simulink library "eng_simple_transient_std"  (Simulink 8.7)
settings: Solver=ode45  StartTime=0.0  StopTime=10.0  RelTol=1e-3
undefined symbols (not defined in the file): DiscIntNeverNeededParam, sMP
libraries: simulink x17
(part 3 of 3)

== system eng_simple_transient_std/eng_simple_transient_std/Airpath_model/Intake flows calculation/EGRTAT filter ==
  EGRTAT_sp : Inport
  Constant : Constant
  Digital Clock : DigitalClock  SampleTime=-1
  Fcn : Fcn  Expr=u(2)/(u(2)+u(1))
  Initialisation : Switch  Criteria=u2 > Threshold
  Lookup Table : Lookup  InputValues=Fiter_calibration_fmode_x_NMOT_rpm  Table=Fiter_calibration_fmode_y_tc_EGRTAT  LookUpMeth=Interpolation-Use End Values
  Memory4 : Memory  InheritSampleTime=on
  Mux : Mux  Inputs=2
  Product : Product  SaturateOnIntegerOverflow=on  InputSameDT=on  OutDataTypeStr=Inherit: Same as first input
  Product1 : Product  SaturateOnIntegerOverflow=on  InputSameDT=on  OutDataTypeStr=Inherit: Same as first input
  Sum : Sum  Inputs=|+-  SaturateOnIntegerOverflow=on  InputSameDT=on  OutDataTypeStr=Inherit: Same as first input
  Sum1 : Sum  Inputs=|++  SaturateOnIntegerOverflow=on  InputSameDT=on  OutDataTypeStr=Inherit: Same as first input
  dt : Constant  Value=Fiter_calibration_dt
  EGRTAT : Outport
  wires:
  Initialisation/1 -> EGRTAT/1, Memory4/1
  Sum1/1 -> Initialisation/1
  Digital Clock/1 -> Initialisation/2
  Fcn/1 -> Sum/2, Product1/1
  Constant/1 -> Sum/1
  Sum/1 -> Product/2
  Product1/1 -> Sum1/2
  Product/1 -> Sum1/1
  Memory4/1 -> Product/1
  EGRTAT_sp/1 -> Initialisation/3, Product1/2
  dt/1 -> Mux/2
  Lookup Table/1 -> Mux/1
  Mux/1 -> Fcn/1
  [EngSpeed] -> Lookup Table/1

== system eng_simple_transient_std/eng_simple_transient_std/Engine_model/AdBlue consumption/Calc_AdBlue_Consumption ==
  brakingMode : Inport
  MAdBlue_kgh : Inport  Port=2
  MAdBlue_braking : Constant  Value=0
  Multiport Switch1 : MultiPortSwitch  DataPortOrder=Zero-based contiguous  Inputs=5  zeroidx=on
  rpm->rph2 : Gain  Gain=1/2
  MAdBlue_brk_kgh : Outport
  wires:
  MAdBlue_kgh/1 -> Multiport Switch1/6, rpm->rph2/1, Multiport Switch1/2
  MAdBlue_braking/1 -> Multiport Switch1/5
  rpm->rph2/1 -> Multiport Switch1/4, Multiport Switch1/3
  brakingMode/1 -> Multiport Switch1/1
  Multiport Switch1/1 -> MAdBlue_brk_kgh/1

== system eng_simple_transient_std/eng_simple_transient_std/Engine_model/Fuel consumption calculation/Calc_Fuel_Flow ==
  brakingMode : Inport
  Mfuel_mgstr_sp : Inport  Port=2
  Constant : Constant  Value=Eng_characteristics_n_cylinder
  Mfuel_Braking : Constant  Value=0
  Multiport Switch1 : MultiPortSwitch  DataPortOrder=Zero-based contiguous  Inputs=5  zeroidx=on
  Product : Product  RndMeth=Zero
  fuelConsumtion_kgh1 : Product  Inputs=**
  mg_str->kg_rota : Fcn  Expr=u/2/1e6
  rpm->rph1 : Gain  Gain=60
  rpm->rph2 : Gain  Gain=1/2
  MFuel_kgh : Outport
  wires:
  Constant/1 -> Product/1
  Product/1 -> mg_str->kg_rota/1
  Multiport Switch1/1 -> Product/2
  Mfuel_mgstr_sp/1 -> Multiport Switch1/6, rpm->rph2/1, Multiport Switch1/2
  rpm->rph1/1 -> fuelConsumtion_kgh1/2
  mg_str->kg_rota/1 -> fuelConsumtion_kgh1/1
  [EngSpeed] -> rpm->rph1/1
  Mfuel_Braking/1 -> Multiport Switch1/5
  rpm->rph2/1 -> Multiport Switch1/4, Multiport Switch1/3
  brakingMode/1 -> Multiport Switch1/1
  fuelConsumtion_kgh1/1 -> MFuel_kgh/1

== system eng_simple_transient_std/eng_simple_transient_std/Engine_model/Fuel consumption calculation/Calc_Fuel_Flow_Consumption ==
  brakingMode : Inport
  Mfuel_mgstr_sp : Inport  Port=2
  Constant : Constant  Value=Eng_characteristics_n_cylinder
  Mfuel_Braking : Constant  Value=0
  Multiport Switch1 : MultiPortSwitch  DataPortOrder=Zero-based contiguous  Inputs=5  zeroidx=on
  Product : Product  RndMeth=Zero
  fuelConsumtion_kgh1 : Product  Inputs=**
  mg_str->kg_rota : Fcn  Expr=u/2/1e6
  rpm->rph1 : Gain  Gain=60
  rpm->rph2 : Gain  Gain=1/2
  MFuel_kgh : Outport
  wires:
  fuelConsumtion_kgh1/1 -> MFuel_kgh/1
  brakingMode/1 -> Multiport Switch1/1
  rpm->rph2/1 -> Multiport Switch1/3, Multiport Switch1/4
  Mfuel_Braking/1 -> Multiport Switch1/5
  [EngSpeed] -> rpm->rph1/1
  mg_str->kg_rota/1 -> fuelConsumtion_kgh1/1
  rpm->rph1/1 -> fuelConsumtion_kgh1/2
  Mfuel_mgstr_sp/1 -> Multiport Switch1/2, rpm->rph2/1, Multiport Switch1/6
  Multiport Switch1/1 -> Product/2
  Product/1 -> mg_str->kg_rota/1
  Constant/1 -> Product/1

== system eng_simple_transient_std/eng_simple_transient_std/Engine_model/Fuel consumption calculation/Calc_Fuel_Flow_TM1_Consumption ==
  brakingMode : Inport
  Mfuel_mgstr_sp : Inport  Port=2
  Constant : Constant  Value=Eng_characteristics_n_cylinder
  Mfuel_Braking : Constant  Value=0
  Multiport Switch1 : MultiPortSwitch  DataPortOrder=Zero-based contiguous  Inputs=5  zeroidx=on
  Product : Product  RndMeth=Zero
  fuelConsumtion_kgh1 : Product  Inputs=**
  mg_str->kg_rota : Fcn  Expr=u/2/1e6
  rpm->rph1 : Gain  Gain=60
  rpm->rph2 : Gain  Gain=1/2
  MFuel_kgh : Outport
  wires:
  Constant/1 -> Product/1
  Product/1 -> mg_str->kg_rota/1
  Multiport Switch1/1 -> Product/2
  Mfuel_mgstr_sp/1 -> Multiport Switch1/6, rpm->rph2/1, Multiport Switch1/2
  rpm->rph1/1 -> fuelConsumtion_kgh1/2
  mg_str->kg_rota/1 -> fuelConsumtion_kgh1/1
  [EngSpeed] -> rpm->rph1/1
  Mfuel_Braking/1 -> Multiport Switch1/5
  rpm->rph2/1 -> Multiport Switch1/4, Multiport Switch1/3
  brakingMode/1 -> Multiport Switch1/1
  fuelConsumtion_kgh1/1 -> MFuel_kgh/1

== system eng_simple_transient_std/eng_simple_transient_std/Engine_model/Fuel consumption calculation/T2N correction ==
  Constant : Constant
  Product : Product  RndMeth=Zero
  Setpoint_fuelledMode_z_dMFueldT2N : Lookup2D  RowIndex=Setpoint_fuelledMode_y_alphaTorque  ColumnIndex=Setpoint_fuelledMode_x_NMOTW_rpm  Table=Setpoint_fuelledMode_z_dMFueldT2N
  Sum : Sum  Inputs=|+-
  Sum1 : Sum  Inputs=|++
  dMFueldT2N : Outport
  wires:
  [T2N_extern] -> Sum/1
  [T2N_degC_sp] -> Sum/2
  [alphaTorque] -> Setpoint_fuelledMode_z_dMFueldT2N/1
  [EngSpeed] -> Setpoint_fuelledMode_z_dMFueldT2N/2
  Setpoint_fuelledMode_z_dMFueldT2N/1 -> Product/1
  Sum/1 -> Product/2
  Product/1 -> Sum1/1
  Constant/1 -> Sum1/2
  Sum1/1 -> dMFueldT2N/1

== system eng_simple_transient_std/eng_simple_transient_std/Engine_model/Fuel consumption calculation/TWE correction ==
  Constant : Constant
  Product : Product  RndMeth=Zero
  Setpoint_fuelledMode_z_dMFueldTWE : Lookup2D  RowIndex=Setpoint_fuelledMode_y_alphaTorque  ColumnIndex=Setpoint_fuelledMode_x_NMOTW_rpm  Table=Setpoint_fuelledMode_z_dMFueldTWE
  Sum : Sum  Inputs=|+-
  Sum1 : Sum  Inputs=|++
  dMFueldTWE : Outport
  wires:
  Sum1/1 -> dMFueldTWE/1
  Constant/1 -> Sum1/2
  Product/1 -> Sum1/1
  Sum/1 -> Product/2
  Setpoint_fuelledMode_z_dMFueldTWE/1 -> Product/1
  [EngSpeed] -> Setpoint_fuelledMode_z_dMFueldTWE/2
  [alphaTorque] -> Setpoint_fuelledMode_z_dMFueldTWE/1
  [TWE_degC_sp] -> Sum/2
  [eng_CoolantEngineIn_Temperature] -> Sum/1

== system eng_simple_transient_std/eng_simple_transient_std/Outputs/Calc_exhGas/rCO2_calc ==
  AFR : Inport
  haluft : Inport  Port=2
  Constant2 : Constant  Value=0.0325
  Constant3 : Constant  Value=1000
  Constant5 : Constant  Value=0.0725
  Gain1 : Gain  Gain=0.5
  MolH1 : Constant  Value=18.01528
  Product1 : Product  Inputs=***//  RndMeth=Zero
  Product2 : Product  Inputs=*/  RndMeth=Zero
  Stoech_coeff : Constant  Value=Eng_characteristics_Stoech_coeff
  Sum1 : Sum  Inputs=3
  CO2_molfrac : Outport
  wires:
  Constant5/1 -> Product2/1
  Sum1/1 -> Product2/2
  Gain1/1 -> Sum1/2
  Constant2/1 -> Sum1/1
  Product1/1 -> Sum1/3
  AFR/1 -> Product1/2, Gain1/1
  Stoech_coeff/1 -> Product1/3
  MolH1/1 -> Product1/5
  Constant3/1 -> Product1/4
  haluft/1 -> Product1/1
  Product2/1 -> CO2_molfrac/1

== system eng_simple_transient_std/eng_simple_transient_std/Outputs/Calc_exhGas/rH2O_calc ==
  AFR : Inport
  haluft : Inport  Port=2
  Constant2 : Constant  Value=0.0325
  Constant3 : Constant  Value=1000
  Constant5 : Constant  Value=0.065
  Gain : Gain  Gain=0.5
  MolH1 : Constant  Value=18.01528
  Product1 : Product  Inputs=***//  RndMeth=Zero
  Product2 : Product  Inputs=*/  RndMeth=Zero
  Stoech_coeff : Constant  Value=Eng_characteristics_Stoech_coeff
  Sum1 : Sum  Inputs=3
  Sum3 : Sum  Inputs=|++
  rH2O_Abg : Outport
  wires:
  Product2/1 -> rH2O_Abg/1
  Constant5/1 -> Sum3/1
  Sum3/1 -> Product2/1
  Sum1/1 -> Product2/2
  Gain/1 -> Sum1/2
  Constant2/1 -> Sum1/1
  Product1/1 -> Sum3/2, Sum1/3
  AFR/1 -> Product1/2, Gain/1
  Stoech_coeff/1 -> Product1/3
  MolH1/1 -> Product1/5
  Constant3/1 -> Product1/4
  haluft/1 -> Product1/1

== system eng_simple_transient_std/eng_simple_transient_std/Outputs/Calc_exhGas/rO2_calc ==
  AFR : Inport
  haluft : Inport  Port=2
  Constant1 : Constant  Value=0.0325
  Constant2 : Constant
  Constant4 : Constant  Value=1000
  Gain1 : Gain  Gain=0.5
  Gain2 : Gain  Gain=0.105
  Lim 0<x<0.2078 => lambda<100 : Saturate  UpperLimit=0.2078376487  LowerLimit=1e-16  LinearizeAsGain=off  ZeroCross=off
  MolH2 : Constant  Value=18.01528
  Product3 : Product  Inputs=***//  RndMeth=Zero
  Product4 : Product  Inputs=*/  RndMeth=Zero
  Stoech_coeff : Constant  Value=Eng_characteristics_Stoech_coeff
  Sum1 : Sum  Inputs=+-
  Sum2 : Sum  Inputs=3
  rO2_Abg : Outport
  wires:
  Product4/1 -> Lim 0<x<0.2078 => lambda<100/1
  Gain2/1 -> Product4/1
  Sum1/1 -> Gain2/1
  Constant2/1 -> Sum1/2
  Sum2/1 -> Product4/2
  Gain1/1 -> Sum2/2
  Constant1/1 -> Sum2/1
  Product3/1 -> Sum2/3
  AFR/1 -> Product3/2, Gain1/1, Sum1/1
  Stoech_coeff/1 -> Product3/3
  MolH2/1 -> Product3/5
  Constant4/1 -> Product3/4
  haluft/1 -> Product3/1
  Lim 0<x<0.2078 => lambda<100/1 -> rO2_Abg/1

== system eng_simple_transient_std/eng_simple_transient_std/SetPoint_model/Starter model/engStarted actualisation ==
  b_ignition : Inport
  Trigger : TriggerPort  VariantControl=Variant
  EngStarted : Outport
  wires:
  b_ignition/1 -> EngStarted/1

== system eng_simple_transient_std/eng_simple_transient_std/SetPoint_model/Starter model/starter torque filter ==
  starterTorque_sp : Inport
  Constant : Constant
  Fcn : Fcn  Expr=u(2)/(u(2)+u(1))
  Memory4 : Memory  InheritSampleTime=on
  Mux : Mux  Inputs=2
  Product : Product  SaturateOnIntegerOverflow=on  InputSameDT=on  OutDataTypeStr=Inherit: Same as first input
  Product1 : Product  SaturateOnIntegerOverflow=on  InputSameDT=on  OutDataTypeStr=Inherit: Same as first input
  Sum : Sum  Inputs=|+-  SaturateOnIntegerOverflow=on  InputSameDT=on  OutDataTypeStr=Inherit: Same as first input
  Sum1 : Sum  Inputs=|++  SaturateOnIntegerOverflow=on  InputSameDT=on  OutDataTypeStr=Inherit: Same as first input
  dt : Constant  Value=Fiter_calibration_dt
  tc starter : Constant  Value=Eng_starter_time_constant
  starterTorque : Outport
  wires:
  tc starter/1 -> Mux/1
  Sum1/1 -> Memory4/1, starterTorque/1
  Fcn/1 -> Sum/2, Product1/1
  Constant/1 -> Sum/1
  Sum/1 -> Product/2
  Product1/1 -> Sum1/2
  Product/1 -> Sum1/1
  Memory4/1 -> Product/1
  starterTorque_sp/1 -> Product1/2
  dt/1 -> Mux/2
  Mux/1 -> Fcn/1

== system eng_simple_transient_std/eng_simple_transient_std/SetPoint_model/Torque setpoint/Alpha_p2s_Br1 calculation ==
  p2s : Inport
  EngSpeed : Inport  Port=2
  Constant : Constant  Value=1e-6
  Divide : Product  Inputs=*/
  MaxBrakingPressure : Lookup2D  RowIndex=Setpoint_brakingMode1_y_alphaTorque  ColumnIndex=Setpoint_brakingMode1_x_NMOTW_rpm  Table=Setpoint_brakingMode1_z_P2S_mbar
  MinBrakingPressure : Lookup2D  RowIndex=Setpoint_brakingMode1_y_alphaTorque  ColumnIndex=Setpoint_brakingMode1_x_NMOTW_rpm  Table=Setpoint_brakingMode1_z_P2S_mbar
  MinMax : MinMax  Function=max  Inputs=2
  Saturation : Saturate  UpperLimit=1  LowerLimit=0
  Subtract : Sum  Inputs=-+
  Subtract1 : Sum  Inputs=+-
  alpha0 : Constant  Value=0
  alpha1 : Constant
  alpha_p2s_br1 : Outport
  wires:
  Saturation/1 -> alpha_p2s_br1/1
  Subtract1/1 -> Divide/1
  MaxBrakingPressure/1 -> Subtract/2
  MinBrakingPressure/1 -> Subtract1/2, Subtract/1
  p2s/1 -> Subtract1/1
  EngSpeed/1 -> MinBrakingPressure/2, MaxBrakingPressure/2
  alpha1/1 -> MaxBrakingPressure/1
  alpha0/1 -> MinBrakingPressure/1
  Divide/1 -> Saturation/1
  Constant/1 -> MinMax/2
  Subtract/1 -> MinMax/1
  MinMax/1 -> Divide/2

== system eng_simple_transient_std/eng_simple_transient_std/SetPoint_model/Torque setpoint/Alpha_p2s_Br2 calculation ==
  p2s : Inport
  EngSpeed : Inport  Port=2
  Constant : Constant  Value=1e-6
  Divide : Product  Inputs=*/
  MaxBrakingPressure : Lookup2D  RowIndex=Setpoint_brakingMode2_y_alphaTorque  ColumnIndex=Setpoint_brakingMode2_x_NMOTW_rpm  Table=Setpoint_brakingMode2_z_P2S_mbar
  MinBrakingPressure : Lookup2D  RowIndex=Setpoint_brakingMode2_y_alphaTorque  ColumnIndex=Setpoint_brakingMode2_x_NMOTW_rpm  Table=Setpoint_brakingMode2_z_P2S_mbar
  MinMax : MinMax  Function=max  Inputs=2
  Saturation : Saturate  UpperLimit=1  LowerLimit=0
  Subtract : Sum  Inputs=-+
  Subtract1 : Sum  Inputs=+-
  alpha0 : Constant  Value=0
  alpha1 : Constant
  alpha_p2s_br2 : Outport
  wires:
  Saturation/1 -> alpha_p2s_br2/1
  Subtract1/1 -> Divide/1
  MaxBrakingPressure/1 -> Subtract/2
  MinBrakingPressure/1 -> Subtract1/2, Subtract/1
  p2s/1 -> Subtract1/1
  EngSpeed/1 -> MinBrakingPressure/2, MaxBrakingPressure/2
  alpha1/1 -> MaxBrakingPressure/1
  alpha0/1 -> MinBrakingPressure/1
  Divide/1 -> Saturation/1
  Constant/1 -> MinMax/2
  Subtract/1 -> MinMax/1
  MinMax/1 -> Divide/2

== system eng_simple_transient_std/eng_simple_transient_std/SetPoint_model/Torque setpoint/Alpha_p2s_Br3 calculation ==
  p2s : Inport
  EngSpeed : Inport  Port=2
  Constant : Constant  Value=1e-6
  Divide : Product  Inputs=*/
  MaxBrakingPressure : Lookup2D  RowIndex=Setpoint_brakingMode3_y_alphaTorque  ColumnIndex=Setpoint_brakingMode3_x_NMOTW_rpm  Table=Setpoint_brakingMode3_z_P2S_mbar
  MinBrakingPressure : Lookup2D  RowIndex=Setpoint_brakingMode3_y_alphaTorque  ColumnIndex=Setpoint_brakingMode3_x_NMOTW_rpm  Table=Setpoint_brakingMode3_z_P2S_mbar
  MinMax : MinMax  Function=max  Inputs=2
  Saturation : Saturate  UpperLimit=1  LowerLimit=0
  Subtract : Sum  Inputs=-+
  Subtract1 : Sum  Inputs=+-
  alpha0 : Constant  Value=0
  alpha1 : Constant
  alpha_p2s_br3 : Outport
  wires:
  Saturation/1 -> alpha_p2s_br3/1
  Subtract1/1 -> Divide/1
  MaxBrakingPressure/1 -> Subtract/2
  MinBrakingPressure/1 -> Subtract1/2, Subtract/1
  p2s/1 -> Subtract1/1
  EngSpeed/1 -> MinBrakingPressure/2, MaxBrakingPressure/2
  alpha1/1 -> MaxBrakingPressure/1
  alpha0/1 -> MinBrakingPressure/1
  Divide/1 -> Saturation/1
  Constant/1 -> MinMax/2
  Subtract/1 -> MinMax/1
  MinMax/1 -> Divide/2

== system eng_simple_transient_std/eng_simple_transient_std/SetPoint_model/alpha torque calculation/AlphaBr1 calculation ==
  mcm_act_braking_trq : Inport
  EngSpeed : Inport  Port=2
  Constant : Constant  Value=-1e-6
  Divide : Product  Inputs=*/
  MaxBrakingTorque : Lookup2D  RowIndex=Setpoint_brakingMode1_y_alphaTorque  ColumnIndex=Setpoint_brakingMode1_x_NMOTW_rpm  Table=Setpoint_brakingMode1_z_Torque_Nm
  MinBrakingTorque : Lookup2D  RowIndex=Setpoint_brakingMode1_y_alphaTorque  ColumnIndex=Setpoint_brakingMode1_x_NMOTW_rpm  Table=Setpoint_brakingMode1_z_Torque_Nm
  MinMax : MinMax  Inputs=2
  Subtract : Sum  Inputs=-+
  Subtract1 : Sum  Inputs=+-
  alpha0 : Constant  Value=0
  alpha1 : Constant
  alpha_br1 : Outport
  wires:
  Subtract1/1 -> Divide/1
  MaxBrakingTorque/1 -> Subtract/2
  MinBrakingTorque/1 -> Subtract1/2, Subtract/1
  mcm_act_braking_trq/1 -> Subtract1/1
  EngSpeed/1 -> MinBrakingTorque/2, MaxBrakingTorque/2
  alpha1/1 -> MaxBrakingTorque/1
  alpha0/1 -> MinBrakingTorque/1
  Divide/1 -> alpha_br1/1
  Subtract/1 -> MinMax/1
  Constant/1 -> MinMax/2
  MinMax/1 -> Divide/2

== system eng_simple_transient_std/eng_simple_transient_std/SetPoint_model/alpha torque calculation/AlphaBr2 calculation ==
  mcm_act_braking_trq : Inport
  EngSpeed : Inport  Port=2
  Constant : Constant  Value=-1e-6
  Divide : Product  Inputs=*/
  MaxBrakingTorque : Lookup2D  RowIndex=Setpoint_brakingMode2_y_alphaTorque  ColumnIndex=Setpoint_brakingMode2_x_NMOTW_rpm  Table=Setpoint_brakingMode2_z_Torque_Nm
  MinBrakingTorque : Lookup2D  RowIndex=Setpoint_brakingMode2_y_alphaTorque  ColumnIndex=Setpoint_brakingMode2_x_NMOTW_rpm  Table=Setpoint_brakingMode2_z_Torque_Nm
  MinMax : MinMax  Inputs=2
  Subtract : Sum  Inputs=-+
  Subtract1 : Sum  Inputs=+-
  alpha0 : Constant  Value=0
  alpha1 : Constant
  alpha_br2 : Outport
  wires:
  Divide/1 -> alpha_br2/1
  alpha0/1 -> MinBrakingTorque/1
  alpha1/1 -> MaxBrakingTorque/1
  EngSpeed/1 -> MaxBrakingTorque/2, MinBrakingTorque/2
  mcm_act_braking_trq/1 -> Subtract1/1
  MinBrakingTorque/1 -> Subtract/1, Subtract1/2
  MaxBrakingTorque/1 -> Subtract/2
  Subtract1/1 -> Divide/1
  Constant/1 -> MinMax/2
  Subtract/1 -> MinMax/1
  MinMax/1 -> Divide/2

== system eng_simple_transient_std/eng_simple_transient_std/SetPoint_model/alpha torque calculation/AlphaBr3 calculation ==
  mcm_act_braking_trq : Inport
  EngSpeed : Inport  Port=2
  Constant : Constant  Value=-1e-6
  Divide : Product  Inputs=*/
  MaxBrakingTorque : Lookup2D  RowIndex=Setpoint_brakingMode3_y_alphaTorque  ColumnIndex=Setpoint_brakingMode3_x_NMOTW_rpm  Table=Setpoint_brakingMode3_z_Torque_Nm
  MinBrakingTorque : Lookup2D  RowIndex=Setpoint_brakingMode3_y_alphaTorque  ColumnIndex=Setpoint_brakingMode3_x_NMOTW_rpm  Table=Setpoint_brakingMode3_z_Torque_Nm
  MinMax : MinMax  Inputs=2
  Subtract : Sum  Inputs=-+
  Subtract1 : Sum  Inputs=+-
  alpha0 : Constant  Value=0
  alpha1 : Constant
  alpha_br3 : Outport
  wires:
  Divide/1 -> alpha_br3/1
  alpha0/1 -> MinBrakingTorque/1
  alpha1/1 -> MaxBrakingTorque/1
  EngSpeed/1 -> MaxBrakingTorque/2, MinBrakingTorque/2
  mcm_act_braking_trq/1 -> Subtract1/1
  MinBrakingTorque/1 -> Subtract/1, Subtract1/2
  MaxBrakingTorque/1 -> Subtract/2
  Subtract/1 -> MinMax/1
  Subtract1/1 -> Divide/1
  Constant/1 -> MinMax/2
  MinMax/1 -> Divide/2

== system eng_simple_transient_std/eng_simple_transient_std/SetPoint_model/alpha torque calculation/AlphaFm calculation ==
  mcm_trq_act_eff : Inport
  EngSpeed : Inport  Port=2
  Divide : Product  Inputs=*/
  Friction Line : Lookup  InputValues=ECU_torque_x_NMOT_rpm  Table=ECU_torque_y_FrictionLine_MISTEE_Nm
  Full Loqd : Lookup  InputValues=ECU_torque_x_NMOT_rpm  Table=ECU_torque_y_FullLoad_MISTEE_Nm
  Subtract : Sum  Inputs=-+
  Subtract1 : Sum  Inputs=+-
  alpha_fm : Outport
  wires:
  Divide/1 -> alpha_fm/1
  EngSpeed/1 -> Full Loqd/1, Friction Line/1
  mcm_trq_act_eff/1 -> Subtract1/1
  Friction Line/1 -> Subtract/1, Subtract1/2
  Full Loqd/1 -> Subtract/2
  Subtract/1 -> Divide/2
  Subtract1/1 -> Divide/1

== system eng_simple_transient_std/eng_simple_transient_std/SetPoint_model/alpha torque calculation/alpha in engine start ==
  alpha_val : Inport
  mcm_EomEng_Stat_MCM : Inport  Port=2
  EngSpeed : Inport  Port=3
  Switch1 : Switch  Criteria=u2 ~= 0
  alpha torque in start : Gain  Gain=0.4
  engine start : simulink/Logic and Bit Operations/Compare To Constant  relop===  const=2  OutDataTypeStr=uint8
  engine start threshold : simulink/Logic and Bit Operations/Compare To Constant  relop=>=  const=Eng_starter_fuelInj_minEngSpd  OutDataTypeStr=uint8
  alphaTorque : Outport
  wires:
  mcm_EomEng_Stat_MCM/1 -> engine start/1
  engine start/1 -> Switch1/2
  alpha_val/1 -> Switch1/3
  EngSpeed/1 -> engine start threshold/1
  engine start threshold/1 -> alpha torque in start/1
  alpha torque in start/1 -> Switch1/1
  Switch1/1 -> alphaTorque/1
